simulink model "ksrbl_4k4t_hdtrig"  (Simulink 6.2)
settings: Solver=ode45  StartTime=0.0  StopTime=20000  RelTol=1e-3
libraries: xbsIndex_r3 x1214, casper_library x120, xps_library x20
(part 16 of 26)

== system ksrbl_4k4t_hdtrig/pfb_fir_real/pol1_in4_first_tap/pfb_coeff_gen ==
  din : Inport  Port=1  LatchInput=off
  sync : Inport  Port=2  LatchInput=off
  Concat : xbsIndex_r3/Concat  num_inputs=4  explicit_period=off  period=1  dbl_ovrd=off
  Counter : xbsIndex_r3/Counter  cnt_type=Free Running  n_bits=10  bin_pt=0  arith_type=Unsigned  start_count=0  cnt_to=Inf  cnt_by_val=1  operation=Up  explicit_period=on  period=1  load_pin=off  rst=on  en=off  dbl_ovrd=off  show_param=off  use_rpm=on  gen_core=off
      settings: xl_area=[0, 0, 0, 0, 0, 0, 0]
  Delay : xbsIndex_r3/Delay  latency=bram_latency+1  reg_retiming=off  explicit_period=off  period=1  en=off  accept_only_valid=off  init_zero=on  dbl_ovrd=off  show_param=off
      settings: xl_area=[0, 0, 0, 0, 0, 0, 0]
  Delay1 : xbsIndex_r3/Delay  latency=5  reg_retiming=off  explicit_period=off  period=1  en=off  accept_only_valid=off  init_zero=on  dbl_ovrd=off  show_param=off
      settings: xl_area=[0, 0, 0, 0, 0, 0, 0]
  ROM1 : xbsIndex_r3/ROM  depth=1024  initVector=[-2.93076934458067e-005 -6.8418926478008e-005 -0.000107570539924886 -0.000146763813245836 -0.000186000028260302 -0.000225280469100824 -0.000264606422166117 -0.000303979176073857 -0.000343400021613443 -0.000382870251698632 -0.000422391161319945 -0.000461964047497041 -0.000501590209230971 -0.0005412709474562 -0.000581007564992605 -0.000620801366497355 -0.000660653658416545 -0.000700565748936889 -0.000740538947937113 -0.00078057456693934 -0.00082067391906037 -0.000860838318962719 -0.000901069082805661 -0.000941367528196143 -0.000981734974139483 -0.00102217274099007 -0.00106268215040191 -0.00110326452527903 -0.00114392118972581 -0.0011846534689972 -0.00122546268944877 -0.00126635017848677 -0.00130731726451796 -0.0013483652768994 -0.00138949554588815 -0.00143070940259078 -0.00147200817891286 -0.00151339320750837 -0.00155486582172885 -0.00159642735557269 -0.00163807914363408 -0.00167982252105203 -0.00172165882345924 -0.00176358938693085 -0.00180561554793309 -0.00184773864327195 -0.00188996001004155 -0.00193228098557262 -0.0019747029073808 -0.0020172271131148 -0.00205985494050462 -0.00210258772730949 -0.00214542681126588 -0.0021883735300354 -0.00223142922115249 -0.0022745952219722 -0.00231787286961781 -0.00236126350092832 -0.0024047684524059 -0.00244838906016338 -0.00249212665987141 -0.00253598258670578 -0.00257995817529453 -0.00262405475966502 -0.00266827367319098 -0.00271261624853939 -0.00275708381761734 -0.00280167771151886 -0.0028463992604716 -0.00289124979378347 -0.00293623063978932 -0.00298134312579731 -0.00302658857803552 -0.0030719683215982 -0.0031174836803922 -0.00316313597708324 -0.00320892653304201 -0.00325485666829045 -0.00330092770144779 -0.00334714094967656 -0.00339349772862858 -0.00343999935239096 -0.00348664713343185 -0.00353344238254637 -0.00358038640880232 -0.00362748051948589 -0.00367472602004742 -0.00372212421404691 -0.00376967640309967 -0.00381738388682185 -0.0038652479627759 -0.00391326992641603 -0.00396145107103364 -0.00400979268770265 -0.00405829606522486 -0.00410696249007518 -0.00415579324634695 -0.00420478961569713 -0.00425395287729147 -0.00430328430774963 -0.00435278518109039 -0.00440245676867663 -0.00445230033916044 -0.00450231715842815 -0.00455250848954527 -0.00460287559270157 -0.00465341972515591 -0.00470414214118121 -0.00475504409200941 -0.00480612682577624 -0.00485739158746616 -0.00490883961885717 -0.00496047215846563 -0.00501229044149107 -0.00506429569976098 -0.00511648916167559 -0.00516887205215263 -0.00522144559257205 -0.00527421100072079 -0.00532716949073756 -0.00538032227305742 -0.00543367055435663 -0.00548721553749733 -0.00554095842147217 -0.00559490040134908 -0.00564904266821598 -0.0057033864091254 -0.00575793280703929 -0.00581268304077358 -0.005867638284943 -0.00592279970990573 -0.00597816848170811 -0.00603374576202937 -0.00608953270812637 -0.00614553047277829 -0.00620174020423136 -0.00625816304614373 -0.00631480013753008 -0.00637165261270651 -0.00642872160123528 -0.00648600822786963 -0.00654351361249864 -0.00660123887009204 -0.00665918511064505 -0.00671735343912337 -0.00677574495540796 -0.00683436075424006 -0.00689320192516612 -0.00695226955248278 -0.00701156471518188 -0.00707108848689551 -0.00713084193584105 -0.00719082612476632 -0.00725104211089464 -0.00731149094587005 -0.00737217367570251 -0.00743309134071308 -0.00749424497547923 -0.00755563560878018 -0.00761726426354217 -0.00767913195678392 -0.00774123969956206 -0.0078035884969165 -0.00786617934781611 -0.00792901324510418 -0.007992091175444 -0.00805541411926468 -0.00811898305070668 -0.00818279893756764 -0.00824686274124825 -0.00831117541669799 -0.00837573791236119 -0.0084405511701229 -0.00850561612525492 -0.00857093370636201 -0.00863650483532787 -0.00870233042726147 -0.0087684113904433 -0.00883474862627165 -0.00890134302920905 -0.00896819548672877 -0.00903530687926125 -0.00910267808014083 -0.00917030995555227 -0.00923820336447758 -0.00930635915864288 -0.00937477818246512 -0.00944346127299917 -0.00951240925988486 -0.00958162296529397 ...(+16595 chars)]  arith_type="Signed  (2's comp)"  n_bits=8  bin_pt=7  latency=4  init_zero=on  explicit_period=off  period=1  rst=off  init_reg=0  en=off  dbl_ovrd=off  show_param=on  distributed_mem=off  use_rpm=on  gen_core=off
      settings: xl_area=[0, 0, 0, 0, 0, 0, 0]
  ROM2 : xbsIndex_r3/ROM  depth=1024  initVector=[0.000396217603096624 0.000926616538832383 0.00145942741756073 0.00199465227585736 0.00253229312583828 0.00307235195508882 0.00361483072659344 0.00415973137866522 0.00470705582487596 0.00525680595398621 0.00580898362987623 0.00636359069147661 0.00692062895269953 0.0074801002023699 0.00804200620415753 0.00860634869650894 0.00917312939257942 0.00974234998016611 0.0103140121216406 0.0108881174538822 0.0114646675882114 0.0120436641103237 0.0126251085802237 0.0132090025321597 0.0137953474745579 0.014384144889958 0.0149753962349483 0.0155691029401009 0.0161652664099085 0.0167638880227199 0.0173649691306771 0.0179685110596515 0.0185745151091818 0.0191829825524114 0.0197939146360257 0.0204073125801906 0.0210231775784913 0.0216415107978706 0.0222623133785678 0.022885586434059 0.0235113310509961 0.0241395482891474 0.0247702391813372 0.0254034047333876 0.026039045924059 0.0266771637049915 0.0273177590006467 0.0279608327082498 0.0286063856977322 0.0292544188116738 0.0299049328652465 0.0305579286461574 0.0312134069145928 0.0318713684031618 0.0325318138168415 0.033194743832921 0.0338601591009473 0.0345280602426701 0.0351984478519882 0.0358713224948953 0.0365466847094266 0.0372245350056059 0.0379048738653926 0.0385877017426297 0.0392730190629907 0.0399608262239294 0.0406511235946275 0.0413439115159438 0.0420391903003637 0.0427369602319492 0.0434372215662886 0.044139974530447 0.0448452193229172 0.0455529561135711 0.0462631850436111 0.0469759062255217 0.0476911197430224 0.0484088256510201 0.0491290239755618 0.0498517147137886 0.0505768978338891 0.0513045732750538 0.0520347409474291 0.052767400732073 0.0535025524809098 0.054240196016686 0.0549803311329261 0.0557229575938895 0.0564680751345269 0.0572156834604374 0.0579657822478265 0.0587183711434638 0.0594734497646413 0.0602310176991321 0.0609910745051499 0.0617536197113077 0.062518652816579 0.0632861732902563 0.0640561805719136 0.0648286740713662 0.0656036531686326 0.0663811172138965 0.0671610655274689 0.0679434973997506 0.0687284120911955 0.0695158088322738 0.0703056868234362 0.0710980452350778 0.0718928832075028 0.0726901998508896 0.0734899942452566 0.0742922654404273 0.075097012455997 0.0759042342812997 0.076713929875375 0.0775260981669348 0.0783407380543326 0.0791578484055308 0.0799774280580697 0.0807994758190364 0.0816239904650347 0.0824509707421551 0.0832804153659443 0.084112323021377 0.0849466923628268 0.0857835220140373 0.0866228105680947 0.0874645565873998 0.0883087586036414 0.0891554151177692 0.090004524599967 0.0908560854896281 0.0917100961953286 0.0925665550948028 0.093425460534919 0.0942868108316545 0.0951506042700728 0.0960168391042989 0.0968855135574979 0.0977566258218513 0.098630174058536 0.0995061563977013 0.100384570938449 0.101265415748812 0.102148688865734 0.10303438829505 0.103922512011466 0.10481305795854 0.105706024048664 0.106601408163047 0.107499208151694 0.108399421833391 0.109302046995688 0.110207081394882 0.111114522756001 0.112024368772789 0.11293661710769 0.113851265391835 0.114768311225024 0.115687752175718 0.116609585781019 0.117533809546663 0.118460420947004 0.119389417425002 0.120320796392214 0.12125455522878 0.122190691283414 0.123129201873391 0.124070084284544 0.125013335771244 0.125958953556402 0.126906934831452 0.127857276756349 0.128809976459557 0.129765031038045 0.130722437557279 0.131682193051213 0.132644294522291 0.133608738941432 0.134575523248032 0.135544644349957 0.136516099123539 0.137489884413573 0.138465997033314 0.139444433764473 0.140425191357217 0.141408266530165 0.142393655970389 0.143381356333411 0.144371364243204 0.145363676292192 0.14635828904125 0.147355199019706 0.14835440272534 0.149355896624389 0.150359677151549 0.151365740709974 0.152374083671285 0.15338470237557 0.154397593131387 0.155412752215775 0.15643017587425 0.15744986032082 0.158471801737983 0.159495996276738 0.160522440056593 0.161551129165567 0.162582059660204 0.163615227565577 0.1646506288753 0.165688259551532 0.166728115524995 0.167770192694977 0.168814486929346 ...(+14485 chars)]  arith_type="Signed  (2's comp)"  n_bits=8  bin_pt=7  latency=4  init_zero=on  explicit_period=off  period=1  rst=off  init_reg=0  en=off  dbl_ovrd=off  show_param=on  distributed_mem=off  use_rpm=on  gen_core=off
      settings: xl_area=[0, 0, 0, 0, 0, 0, 0]
  ROM3 : xbsIndex_r3/ROM  depth=1024  initVector=[0.999998703172994 0.999993292845694 0.999983662567318 0.999969812430908 0.99995174257015 0.999929453159369 0.999902944413533 0.999872216588243 0.999837269979734 0.999798104924869 0.999754721801137 0.999707121026645 0.999655303060114 0.999599268400876 0.99953901758886 0.999474551204593 0.999405869869187 0.999332974244333 0.999255865032293 0.999174542975888 0.999089008858492 0.998999263504017 0.99890530777691 0.99880714258213 0.998704768865148 0.998598187611927 0.998487399848913 0.998372406643018 0.998253209101611 0.998129808372496 0.998002205643907 0.997870402144482 0.997734399143256 0.997594197949636 0.997449799913391 0.997301206424632 0.99714841891379 0.996991438851602 0.996830267749091 0.996664907157544 0.996495358668494 0.996321623913698 0.996143704565114 0.995961602334884 0.995775318975306 0.995584856278814 0.995390216077955 0.995191400245362 0.994988410693735 0.994781249375808 0.994569918284331 0.994354419452041 0.994134754951632 0.993910926895733 0.993682937436881 0.993450788767484 0.993214483119805 0.992974022765922 0.992729410017703 0.992480647226776 0.992227736784498 0.991970681121922 0.991709482709766 0.991444144058384 0.991174667717725 0.990901056277309 0.990623312366187 0.990341438652908 0.990055437845487 0.989765312691363 0.989471065977372 0.989172700529702 0.98887021921386 0.988563624934636 0.988252920636063 0.987938109301376 0.987619193952979 0.987296177652399 0.986969063500253 0.9866378546362 0.986302554238906 0.985963165525997 0.985619691754023 0.985272136218411 0.984920502253422 0.98456479323211 0.984205012566277 0.983841163706425 0.983473250141718 0.98310127539993 0.9827252430474 0.982345156688988 0.981961019968026 0.981572836566271 0.981180610203857 0.980784344639244 0.980384043669174 0.979979711128617 0.979571350890721 0.979158966866766 0.978742563006105 0.978322143296121 0.97789771176217 0.977469272467528 0.977036829513341 0.976600387038569 0.976159949219934 0.975715520271862 0.975267104446433 0.97481470603332 0.974358329359739 0.973897978790388 0.973433658727389 0.972965373610236 0.972493127915735 0.972016926157941 0.971536772888105 0.971052672694612 0.970564630202924 0.970072650075512 0.969576737011806 0.969076895748125 0.96857313105762 0.96806544775021 0.967553850672519 0.967038344707813 0.96651893477594 0.965995625833259 0.965468422872581 0.964937330923102 0.964402355050338 0.963863500356057 0.963320771978216 0.962774175090892 0.962223714904214 0.961669396664297 0.961111225653173 0.960549207188721 0.9599833466246 0.959413649350177 0.958840120790461 0.958262766406025 0.957681591692943 0.957096602182714 0.95650780344219 0.955915201073506 0.955318800714006 0.954718608036168 0.954114628747533 0.953506868590629 0.952895333342897 0.952280028816617 0.95166096085883 0.951038135351263 0.950411558210255 0.949781235386675 0.949147172865852 0.94850937666749 0.947867852845593 0.947222607488389 0.946573646718244 0.945920976691592 0.945264603598845 0.944604533664322 0.94394077314616 0.94327332833624 0.9426022055601 0.941927411176856 0.941248951579118 0.940566833192909 0.939881062477578 0.93919164592572 0.938498590063092 0.937801901448525 0.937101586673841 0.936397652363768 0.935690105175855 0.934978951800382 0.934264198960279 0.933545853411033 0.932823921940605 0.932098411369339 0.931369328549878 0.93063668036707 0.929900473737883 0.929160715611313 0.928417412968295 0.927670572821616 0.926920202215816 0.926166308227106 0.925408897963271 0.924647978563581 0.923883557198696 0.923115641070577 0.922344237412387 0.921569353488406 0.920790996593929 0.920009174055177 0.919223893229202 0.918435161503787 0.917642986297359 0.916847375058886 0.916048335267785 0.915245874433821 0.914440000097018 0.913630719827555 0.912818041225669 0.91200197192156 0.911182519575291 0.910359691876691 0.909533496545251 0.908703941330029 0.907871034009552 0.907034782391709 0.906195194313657 0.905352277641716 0.90450604027127 0.903656490126664 0.902803635161105 0.901947483356553 0.901088042723628 0.900225321301497 0.899359327157778 ...(+14480 chars)]  arith_type="Signed  (2's comp)"  n_bits=8  bin_pt=7  latency=4  init_zero=on  explicit_period=off  period=1  rst=off  init_reg=0  en=off  dbl_ovrd=off  show_param=off  distributed_mem=off  use_rpm=on  gen_core=off
      settings: xl_area=[0, 0, 0, 0, 0, 0, 0]
  ROM4 : xbsIndex_r3/ROM  depth=1024  initVector=[-0.000394733804378599 -0.00091894009097766 -0.00144074209396071 -0.00196014196092343 -0.00247714186351929 -0.00299174399738666 -0.0035039505820764 -0.00401376386097833 -0.00452118610124794 -0.00502621959373242 -0.00552886665289705 -0.00602912961675077 -0.00652701084677175 -0.00702251272783237 -0.00751563766812467 -0.00800638809908481 -0.00849476647531741 -0.00898077527452013 -0.0094644169974074 -0.00994569416763431 -0.0104246093317198 -0.0109011650589701 -0.011375363941402 -0.011847208593665 -0.0123167016529641 -0.0127838457789822 -0.013248643653802 -0.0137110979818276 -0.0141712114897063 -0.01462898692625 -0.015084427062356 -0.0155375346909277 -0.0159883126267958 -0.0164367637066384 -0.016882890788901 -0.0173266967537165 -0.0177681845028252 -0.0182073569594939 -0.0186442170684354 -0.0190787677957276 -0.0195110121287322 -0.0199409530760134 -0.020368593667256 -0.0207939369531843 -0.0212169860054792 -0.0216377439166969 -0.0220562138001854 -0.0224723987900028 -0.0228863020408342 -0.023297926727908 -0.0237072760469137 -0.0241143532139177 -0.0245191614652799 -0.0249217040575696 -0.025321984267482 -0.0257200053917533 -0.0261157707470769 -0.0265092836700182 -0.0269005475169301 -0.0272895656638681 -0.0276763415065047 -0.0280608784600444 -0.0284431799591382 -0.0288232494577974 -0.029201090429308 -0.0295767063661448 -0.0299501007798847 -0.0303212772011205 -0.0306902391793742 -0.0310569902830104 -0.031421534099149 -0.0317838742335783 -0.0321440143106675 -0.0325019579732798 -0.0328577088826839 -0.0332112707184669 -0.0335626471784461 -0.0339118419785808 -0.0342588588528843 -0.0346037015533351 -0.0349463738497889 -0.0352868795298891 -0.0356252223989786 -0.0359614062800104 -0.0362954350134587 -0.0366273124572291 -0.0369570424865697 -0.0372846289939812 -0.0376100758891271 -0.0379333870987439 -0.0382545665665512 -0.0385736182531612 -0.0388905461359889 -0.0392053542091611 -0.0395180464834262 -0.0398286269860635 -0.0401370997607924 -0.040443468867681 -0.0407477383830558 -0.04104991239941 -0.041349995025312 -0.0416479903853147 -0.0419439026198631 -0.0422377358852034 -0.0425294943532907 -0.042819182211697 -0.0431068036635199 -0.0433923629272899 -0.0436758642368781 -0.0439573118414042 -0.0442367100051441 -0.0445140630074369 -0.0447893751425929 -0.0450626507198003 -0.0453338940630326 -0.0456031095109556 -0.0458703014168347 -0.0461354741484411 -0.0463986320879593 -0.0466597796318932 -0.0469189211909733 -0.0471760611900625 -0.0474312040680633 -0.0476843542778235 -0.0479355162860429 -0.0481846945731794 -0.0484318936333548 -0.0486771179742614 -0.0489203721170673 -0.0491616605963231 -0.0494009879598667 -0.0496383587687299 -0.0498737775970439 -0.0501072490319443 -0.0503387776734775 -0.0505683681345058 -0.0507960250406126 -0.051021753030008 -0.0512455567534343 -0.0514674408740707 -0.051687410067439 -0.0519054690213085 -0.052121622435601 -0.0523358750222962 -0.052548231505336 -0.0527586966205303 -0.0529672751154612 -0.0531739717493881 -0.0533787912931527 -0.0535817385290833 -0.0537828182509 -0.053982035263619 -0.0541793943834576 -0.0543749004377385 -0.0545685582647947 -0.0547603727138737 -0.0549503486450423 -0.055138490929091 -0.0553248044474387 -0.0555092940920366 -0.0556919647652731 -0.0558728213798782 -0.0560518688588276 -0.0562291121352474 -0.056404556152318 -0.056578205863179 -0.0567500662308333 -0.056920142228051 -0.0570884388372744 -0.057254961050522 -0.0574197138692925 -0.0575827023044697 -0.0577439313762261 -0.0579034061139279 -0.0580611315560386 -0.0582171127500238 -0.0583713547522553 -0.0585238626279151 -0.0586746414509005 -0.0588236963037274 -0.0589710322774357 -0.0591166544714924 -0.0592605679936971 -0.0594027779600858 -0.0595432894948353 -0.0596821077301675 -0.0598192378062542 -0.0599546848711213 -0.0600884540805531 -0.060220550597997 -0.0603509795944681 -0.0604797462484536 -0.0606068557458172 -0.0607323132797039 -0.0608561240504448 -0.0609782932654615 -0.0610988261391706 -0.0612177278928892 -0.0613350037547389 -0.0614506589595508 ...(+16627 chars)]  arith_type="Signed  (2's comp)"  n_bits=8  bin_pt=7  latency=4  init_zero=on  explicit_period=off  period=1  rst=off  init_reg=0  en=off  dbl_ovrd=off  show_param=off  distributed_mem=off  use_rpm=on  gen_core=off
      settings: xl_area=[0, 0, 0, 0, 0, 0, 0]
  Register : xbsIndex_r3/Register  init=0  reg_only_valid=off  explicit_period=off  period=1  rst=off  en=off  out_en=off  dbl_ovrd=off  show_param=off
      settings: xl_area=[0, 0, 0, 0, 0, 0, 0]
  Reinterpret{1..4} (4 alike) : xbsIndex_r3/Reinterpret  force_arith_type=on  arith_type=Unsigned  force_bin_pt=on  bin_pt=0  force_valid=on
  dout : Outport
  sync_out : Outport  Port=2
  coeff : Outport  Port=3
  wires:
  din/1 -> Delay1/1
  Delay1/1 -> dout/1
  sync/1 -> Counter/1, Delay/1
  Delay/1 -> sync_out/1
  Concat/1 -> Register/1
  Register/1 -> coeff/1
  Counter/1 -> ROM1/1, ROM2/1, ROM3/1, ROM4/1
  ROM1/1 -> Reinterpret1/1
  Reinterpret1/1 -> Concat/1
  ROM2/1 -> Reinterpret2/1
  Reinterpret2/1 -> Concat/2
  ROM3/1 -> Reinterpret3/1
  Reinterpret3/1 -> Concat/3
  ROM4/1 -> Reinterpret4/1
  Reinterpret4/1 -> Concat/4
